simulink model "rowFaz_schemat"  (R2024b)
settings: Solver=VariableStepAuto  StartTime=0.0  StopTime=10.0  MaxStep=0.05  RelTol=1e-3
undefined symbols (not defined in the file): czas_skok, dU, ksi, U0, wn, X0, Xp0
settings Model: Creator=Michal  LastModifiedBy=Michal
settings DataIOCC: ReturnWorkspaceOutputs=off

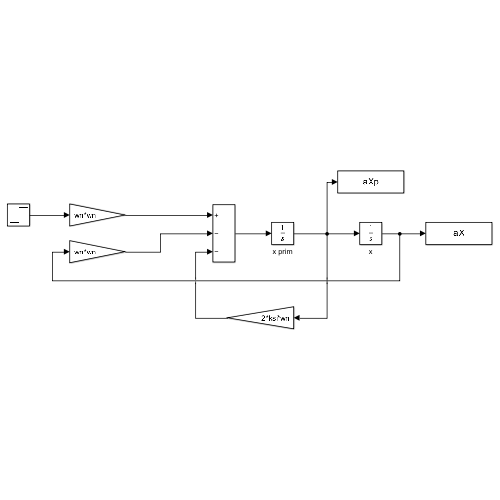
[thumbnail: Simulink's stored preview of the top-level diagram]
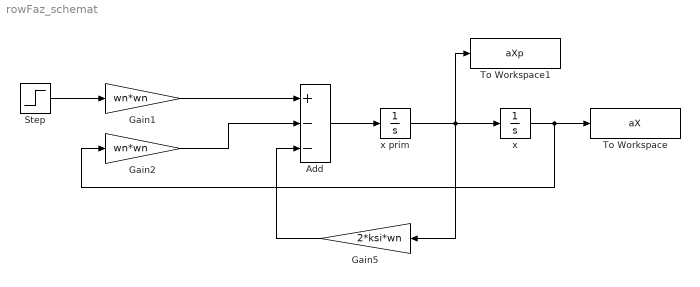
== system rowFaz_schemat ==
  Add : Sum  Inputs=+--
  Gain1 : Gain  Gain=wn*wn
  Gain2 : Gain  Gain=wn*wn
  Gain5 : Gain  Gain=2*ksi*wn
  Step : Step  Time=czas_skok  Before=U0  After=U0+dU  SampleTime=0
  To Workspace : ToWorkspace  VariableName=aX  SampleTime=-1
  To Workspace1 : ToWorkspace  VariableName=aXp  SampleTime=-1
  x : Integrator  InitialCondition=X0
  x prim : Integrator  InitialCondition=Xp0
  wires:
  x prim/1 -> To Workspace1/1, Gain5/1, x/1
  Step/1 -> Gain1/1
  Add/1 -> x prim/1
  x/1 -> Gain2/1, To Workspace/1
  Gain5/1 -> Add/3
  Gain2/1 -> Add/2
  Gain1/1 -> Add/1
